simulink library "AEMACE8_OUT"  (R2021b)
settings: Solver=VariableStepAuto  StartTime=0.0  StopTime=10.0  RelTol=1e-3
settings Model: Creator=ACH  LastModifiedBy=C83127

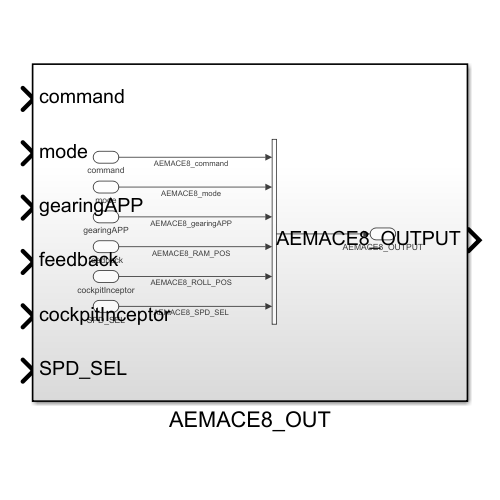
[thumbnail: Simulink's stored preview of the top-level diagram]
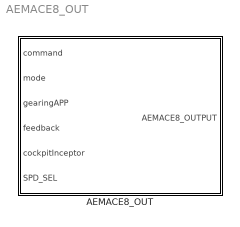
== system AEMACE8_OUT ==
  AEMACE8_OUT : Subsystem

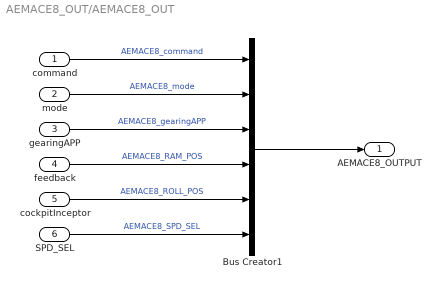
== system AEMACE8_OUT/AEMACE8_OUT ==
  command : Inport
  mode : Inport  Port=2
  gearingAPP : Inport  Port=3
  feedback : Inport  Port=4
  cockpitInceptor : Inport  Port=5
  SPD_SEL : Inport  Port=6
  Bus Creator1 : BusCreator  Inputs=6  OutDataTypeStr=Bus: AEMACE8_OUTPUT
  AEMACE8_OUTPUT : Outport  OutDataTypeStr=Bus: AEMACE8_OUTPUT
  wires:
  command/1 -> Bus Creator1/1  "AEMACE8_command"
  mode/1 -> Bus Creator1/2  "AEMACE8_mode"
  Bus Creator1/1 -> AEMACE8_OUTPUT/1
  gearingAPP/1 -> Bus Creator1/3  "AEMACE8_gearingAPP"
  feedback/1 -> Bus Creator1/4  "AEMACE8_RAM_POS"
  cockpitInceptor/1 -> Bus Creator1/5  "AEMACE8_ROLL_POS"
  SPD_SEL/1 -> Bus Creator1/6  "AEMACE8_SPD_SEL"
